simulink model "adap"  (R2012b)
settings: Solver=ode45  StartTime=0.0  StopTime=10  FixedStep=0.01  RelTol=1e-3
settings Model: Creator=Administrator  LastModifiedBy=Administrator

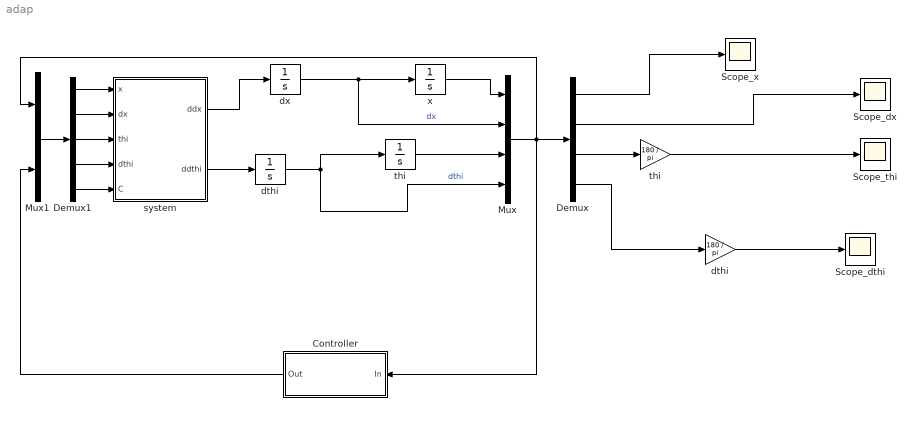
== system adap ==
  Controller : Subsystem  TreatAsAtomicUnit=on
  Demux : Demux
  Demux1 : Demux  Outputs=5
  Mux : Mux
  Mux1 : Mux  Inputs=2
  Scope_dthi : Scope
      settings: SaveName=ScopeData3
  Scope_dx : Scope
  Scope_thi : Scope
      settings: SaveName=ScopeData2
  Scope_x : Scope
  dthi : Integrator
  "dthi " : Gain  Gain=180 / pi
  dx : Integrator
  system : MATLAB Function  TreatAsAtomicUnit=on
  thi : Integrator  InitialCondition=15 * pi / 180
  "thi " : Gain  Gain=180 / pi
  x : Integrator
  wires:
  system/1(ddx) -> dx/1
  dx/1 -> Mux/2, x/1  "dx"
  system/2(ddthi) -> dthi/1
  dthi/1 -> Mux/4, thi/1  "dthi"
  x/1 -> Mux/1
  thi/1 -> Mux/3
  Mux/1 -> Controller/1(In), Demux/1, Mux1/1
  Demux1/5 -> system/5(C)
  Demux1/4 -> system/4(dthi)
  Demux1/3 -> system/3(thi)
  Demux1/2 -> system/2(dx)
  Demux1/1 -> system/1(x)
  Mux1/1 -> Demux1/1
  Demux/3 -> "thi "/1
  Demux/4 -> "dthi "/1
  Demux/1 -> Scope_x/1
  Demux/2 -> Scope_dx/1
  "thi "/1 -> Scope_thi/1
  "dthi "/1 -> Scope_dthi/1
  Controller/1(Out) -> Mux1/2

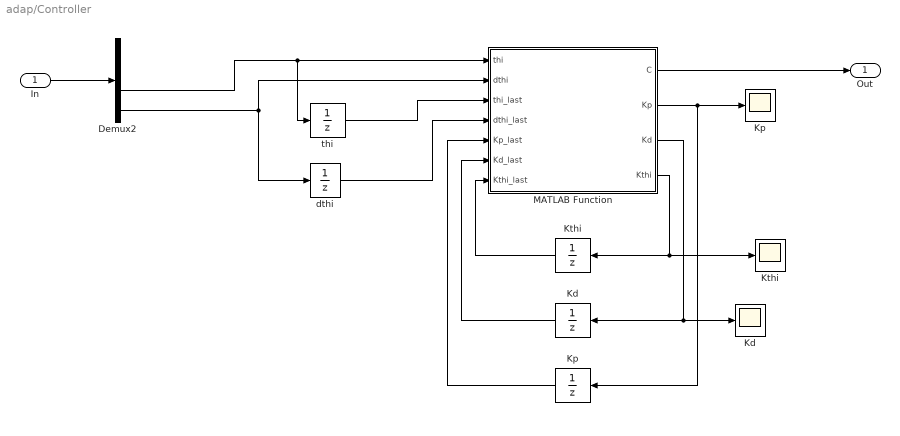
== system adap/Controller ==
  In : Inport
  "   Kp " : UnitDelay  InitialCondition=-24720  SampleTime=0.01
  "  Kd " : UnitDelay  InitialCondition=-3218  SampleTime=0.01
  Demux2 : Demux
  Kd : Scope
      settings: SaveName=ScopeData5
  Kp : Scope
      settings: SaveName=ScopeData4
  Kthi : Scope
      settings: SaveName=ScopeData6
  "Kthi " : UnitDelay  InitialCondition=10  SampleTime=0.01
  MATLAB Function : MATLAB Function  TreatAsAtomicUnit=on
  dthi : UnitDelay  SampleTime=0.01
  thi : UnitDelay  SampleTime=0.01
  Out : Outport
  wires:
  In/1 -> Demux2/1
  MATLAB Function/4(Kthi) -> Kthi/1, "Kthi "/1
  "Kthi "/1 -> MATLAB Function/7(Kthi_last)
  MATLAB Function/3(Kd) -> Kd/1, "  Kd "/1
  "  Kd "/1 -> MATLAB Function/6(Kd_last)
  MATLAB Function/2(Kp) -> "   Kp "/1, Kp/1
  "   Kp "/1 -> MATLAB Function/5(Kp_last)
  Demux2/3 -> thi/1, MATLAB Function/1(thi)
  Demux2/4 -> MATLAB Function/2(dthi), dthi/1
  thi/1 -> MATLAB Function/3(thi_last)
  dthi/1 -> MATLAB Function/4(dthi_last)
  MATLAB Function/1(C) -> Out/1

== matlab function adap/Controller/MATLAB Function ==
  data: thi input; C output; dthi input; thi_last input; dthi_last input; Kp_last input; Kd_last input; Kp output; Kd output; Kthi_last input; Kthi output
function [C, Kp, Kd, Kthi] = fcn(thi, dthi, thi_last, dthi_last, Kp_last, Kd_last, Kthi_last)
wn = 10;
ksi = 0.707;
gama1 = -4;
gama2 = -4;
P = [(ksi / wn) + ((wn ^ 2 + 1) / (4 * ksi))     1 / (2 * wn ^ 2); ...
    1 / (2 * wn ^ 2)                             (wn ^ 2 + 1) / (4 * ksi * wn ^ 3)];
T = [0 0;thi dthi];
T_last = [0 0;thi_last dthi_last];
X = [thi;dthi];
X_last = [thi_last;dthi_last];
A_last = [Kp_last;Kd_last];
A = A_last + 0.5 * gama1 * 0.01 * (T_last' * P * X_last + T' * P * X);
Kp = A(1);
Kd = A(2);
Kthi = Kthi_last + 0.01 * gama2 * ...
    abs(thi / (2 * wn ^ 2) + dthi * (wn ^ 2 + 1) / (4 * ksi * wn ^ 3));
u = -Kthi * sign(thi / (2 * wn ^ 2) + dthi * (wn ^ 2 + 1) / (4 * ksi * wn ^ 3));
C = -Kp * thi - Kd * dthi + u;
end

== matlab function adap/system ==
  data: x input; ddx output; dx input; thi input; dthi input; C input; ddthi output
function [ddx,ddthi] = fcn(x,dx,thi,dthi,C)
Mp = 200;
Mr = 5.5;
D = 0.6;
L = 1;
b = 0.03;
R = 0.2;
Jp = 27.6;
Jr = 0.11;
g = 9.8;
%**************************************************************************
%非线性模型
%**************************************************************************
alpha = Mr * R ^ 2 / Jr + 1;
beta = Jp / (Mp * L * cos(thi)) + L * cos(thi);
gama = L * Mp * g;
A22 = -R ^ 2 * b / (alpha * Jr);
A23 = -R ^ 2 * (gama - Jp * dthi ^ 2 / cos(thi)) / (2 * Jr * alpha * beta);
B2 = R / (2 * Jr) * (1 / alpha + R / (alpha * beta));
A43 = gama / Jp - (L * (gama * cos(thi) - Jp * dthi ^ 2) / (Jp * beta));
B4 = (L * cos(thi) / beta - 1) / Jp;

f2 = 0.5;
f4 = 3;

ddx = A22 * dx + A23 * sin(thi) + B2 * C + f2;
ddthi = A43 * sin(thi) + B4 * C + f4;
